simulink model "IEEE34_SPSload"  (R2021b)
settings: Solver=ode4  StartTime=0.0  StopTime=5  FixedStep=50e-6  RelTol=1e-3
PreLoadFcn:
  | pGain = 0.05; % Gain of random perturbation (pu)
  | pGainAP = 0.01; % Gain of sinusoidal active power variation (pu)
  | pGainRP = 0.01; % Gain of sinusoidal reactive power variation (pu)
  | pFreqAP = 0.03; % Frequency of sinusoidal active power variation (Hz)
  | pFreqRP = 0.03; % Frequency of sinusoidal reactive power variation (Hz)
  | 
  | init_IEEE34nodetestfeeder;
InitFcn:
  | pGain = 0.05; % Gain of random perturbation (pu)
  | pGainAP = 0.01; % Gain of sinusoidal active power variation (pu)
  | pGainRP = 0.01; % Gain of sinusoidal reactive power variation (pu)
  | pFreqAP = 0.03; % Frequency of sinusoidal active power variation (Hz)
  | pFreqRP = 0.03; % Frequency of sinusoidal reactive power variation (Hz)
  | 
  | init_IEEE34nodetestfeeder;
values from neighbouring files (symbols this model uses):
  fNom = f    (= 60)    [init_IEEE34nodetestfeeder.m]
  loadcoeff = 1.0    (= 1)    [init_IEEE34nodetestfeeder.m]
  Ts = 50e-6    (= 5e-05)    [init_IEEE34nodetestfeeder.m]
  vNomMV = VsubL    (= 24900)    [init_IEEE34nodetestfeeder.m]
  VsubL = 24.9e3    (= 24900)    [init_IEEE34nodetestfeeder.m]
  VxfmL = 4.16e3    (= 4160)    [init_IEEE34nodetestfeeder.m]
undefined symbols (not defined in the file or in its folder): Ac, Bc, Cc, Dc, find_system, j
libraries: spsSeriesRLCBranchLib x418, spsGroundLib x242, simulink_extras x176, spsVoltageMeasurementLib x106, spsRMSLib x96, spsControlledCurrentSourceLib x94, spsThreePhaseVIMeasurementLib x37, spsMutualInductanceLib x24, spsCurrentMeasurementLib x12, spsOnDelayLib x12, spsLinearTransformerLib x6, spsControlledVoltageSourceLib x6
(part 18 of 33)

== system IEEE34_SPSload/SM_IEEE34/DL_802-1/Load B1/model/PLL ==
  v (pu) : Inport
  freq (pu) : Inport  Port=2
  Gain : Gain  Gain=2*pi
  Gain1 : Gain  Gain=500
  Gain2 : Gain  Gain=freq
  IC : InitialCondition
  Integrator : Integrator
  Integrator1 : Integrator
  Product : Product  Inputs=**  RndMeth=Zero
  Sum1 : Sum  InputSameDT=on  SaturateOnIntegerOverflow=on  OutDataTypeStr=Inherit: Same as first input
  Trigonometric Function : Trigonometry  Operator=cos
  adaptive filter : Subsystem
  adaptive mean : Subsystem
  alpha (rad) : Outport  VectorParamsAs1DForOutWhenUnconnected=off
  wt : Outport  Port=2  VectorParamsAs1DForOutWhenUnconnected=off
  wires:
  freq (pu)/1 -> Gain2/1
  Gain2/1 -> adaptive filter/2(freq (Hz)), adaptive mean/2(freq (Hz)), Gain/1
  Trigonometric Function/1 -> Product/2
  adaptive mean/1(y) -> alpha (rad)/1
  Integrator1/1 -> Gain1/1
  Gain1/1 -> Sum1/1, adaptive mean/1(u)
  Sum1/1 -> Trigonometric Function/1
  Integrator/1 -> Sum1/2, wt/1
  Gain/1 -> Integrator/1
  adaptive filter/1(y) -> Integrator1/1
  Product/1 -> adaptive filter/1(u)
  v (pu)/1 -> IC/1
  IC/1 -> Product/1

== system IEEE34_SPSload/SM_IEEE34/DL_802-1/Load B1/model/Positive Sequence current ==
  note: kp=Vmin^(np-2)/Vo^np
      | kq=Vmin^(nq-2)/Vo^nq
  note: V<Vmin
      | Constant impedance load :
      |
      |  P=Po*kp*V^2
      | Q=Qo*kq*V^2
  note: V>Vmin :
      |
      |    P=Po*(V/Vo)^np
      |    Q=Qo*(V/Vo)^np
  note: I1= (S/V1)'
  V1(pu) : Inport
  S_ext : Inport  Port=2
  Complex to Magnitude-Angle : ComplexToMagnitudeAngle  Output=Magnitude
  Complex to Real-Imag1 : ComplexToRealImag
  Conj1 : Math  Operator=conj  SignedPower=on  SaturateOnIntegerOverflow=on
  Math Function : Math  Operator=square  SignedPower=on  SaturateOnIntegerOverflow=on
  Mux1 : Mux  Inputs=3
  Mux2 : Mux  Inputs=2
  Mux3 : Mux  Inputs=2
  P0/ (Vo^np) : Gain  Gain=P0/(Mag_V0^np)  SaturateOnIntegerOverflow=on  OutDataTypeStr=Inherit: Same as input  ParamDataTypeStr=Inherit: Same as input
  PQ_ext : Constant  Value=PQext
  Product : Product  Inputs=/*  InputSameDT=on  SaturateOnIntegerOverflow=on  OutDataTypeStr=Inherit: Same as first input
  Q0/(Vo^nq) : Gain  Gain=Q0/(Mag_V0^nq)  SaturateOnIntegerOverflow=on  OutDataTypeStr=Inherit: Same as input  ParamDataTypeStr=Inherit: Same as input
  Real-Imag to Complex : RealImagToComplex
  Switch1 : Switch  Threshold=0.5  InputSameDT=on
  Switch3 : Switch  Threshold=Vmin  InputSameDT=on
  Switch4 : Switch  Threshold=Vmin  InputSameDT=on
  TF_P : Subsystem  mask(Transfer function){T1=Tp1, T2=Tp2, V_Init=P0}
      mask prompts: T1 "Time constant T1 (s):"; T2 "Time constant T2 (s):"; V_Init "Initial input and output :"
      mask help:
      | This block implements a continuous transfer function:
      |
      |          1+T1s
      | H(s)= ------
      |          1+T2s
      |
      | States are initialized according to  initial input and output value so that simulation starts in steady state.
      mask init:
      | numc=[T1 1];
      | denc=[T2 1];
      | [Ac,Bc,Cc,Dc]=tf2ss(numc,denc);
      | 
      | % Compute Initial states
      | I=eye(size(Ac));
      | x0c=inv(-Ac)*Bc*V_Init;
      mask Display: disp('1+T1s\n---\n1+T2s')
  TF_Q : Subsystem  mask(Transfer function){T1=Tq1, T2=Tq2, V_Init=Q0}
      mask prompts: T1 "Time constant T1 (s):"; T2 "Time constant T2 (s):"; V_Init "Initial input and output :"
      mask help:
      | This block implements a continuous transfer function:
      |
      |          1+T1s
      | H(s)= ------
      |          1+T2s
      |
      | States are initialized according to  initial input and output value so that simulation starts in steady state.
      mask init:
      | numc=[T1 1];
      | denc=[T2 1];
      | [Ac,Bc,Cc,Dc]=tf2ss(numc,denc);
      | 
      | % Compute Initial states
      | I=eye(size(Ac));
      | x0c=inv(-Ac)*Bc*V_Init;
      mask Display: disp('1+T1s\n---\n1+T2s')
  V^nq : Fcn  Expr=u[1]^u[2]
  V^nq , : Fcn  Expr=u[1]^u[2]
  Vmin^(np-2) : Gain  Gain=Vmin^(np-2)  SaturateOnIntegerOverflow=on  OutDataTypeStr=Inherit: Same as input  ParamDataTypeStr=Inherit: Same as input
  Vmin^(nq-2) : Gain  Gain=Vmin^(nq-2)  SaturateOnIntegerOverflow=on  OutDataTypeStr=Inherit: Same as input  ParamDataTypeStr=Inherit: Same as input
  np : Constant  Value=np
  nq : Constant  Value=nq
  pu>V : Gain  Gain=Vnom/sqrt(2)  SaturateOnIntegerOverflow=on  OutDataTypeStr=Inherit: Same as input  ParamDataTypeStr=Inherit: Same as input
  I1(A) : Outport  VectorParamsAs1DForOutWhenUnconnected=off
  VPQ : Outport  Port=2  VectorParamsAs1DForOutWhenUnconnected=off
  wires:
  Vmin^(nq-2)/1 -> Switch4/3
  V^nq ,/1 -> Switch3/1
  Vmin^(np-2)/1 -> Switch3/3
  Math Function/1 -> Vmin^(nq-2)/1, Vmin^(np-2)/1
  V^nq/1 -> Switch4/1
  V1(pu)/1 -> Complex to Magnitude-Angle/1, pu>V/1
  Mux3/1 -> V^nq/1
  nq/1 -> Mux3/2
  Mux2/1 -> V^nq ,/1
  np/1 -> Mux2/2
  Switch3/1 -> P0/ (Vo^np)/1
  Q0/(Vo^nq)/1 -> TF_Q/1(In1)
  P0/ (Vo^np)/1 -> TF_P/1(In1)
  Switch4/1 -> Q0/(Vo^nq)/1
  Product/1 -> Conj1/1
  Conj1/1 -> I1(A)/1
  Switch1/1 -> Product/2, Complex to Real-Imag1/1  "S=P+jQ"
  Real-Imag to Complex/1 -> Switch1/3  "S_dyn"
  S_ext/1 -> Switch1/1
  PQ_ext/1 -> Switch1/2
  pu>V/1 -> Product/1
  Complex to Magnitude-Angle/1 -> Math Function/1, Mux3/1, Mux2/1, Switch3/2, Switch4/2, Mux1/1
  Mux1/1 -> VPQ/1
  Complex to Real-Imag1/1 -> Mux1/2
  Complex to Real-Imag1/2 -> Mux1/3
  TF_P/1(Out1) -> Real-Imag to Complex/1
  TF_Q/1(Out1) -> Real-Imag to Complex/2

== system IEEE34_SPSload/SM_IEEE34/DL_802-1/Load C/model/Break Alg. Loop ==
  In : Inport
  Complex to Real-Imag : ComplexToRealImag
  Real-Imag to Complex : RealImagToComplex
  imag : simulink_extras/Additional Linear/Transfer Fcn (with initial outputs)  N=[1]  D="[100e-6  1]"  Y0=imag(I1_init*exp(-j*Pha_V0*pi/180))  U0=imag(I1_init*exp(-j*Pha_V0*pi/180))
  real : simulink_extras/Additional Linear/Transfer Fcn (with initial outputs)  N=[1]  D="[100e-6  1]"  Y0=real(I1_init*exp(-j*Pha_V0*pi/180))  U0=real(I1_init*exp(-j*Pha_V0*pi/180))
  Out : Outport  VectorParamsAs1DForOutWhenUnconnected=off
  wires:
  imag/1 -> Real-Imag to Complex/2
  Complex to Real-Imag/2 -> imag/1
  real/1 -> Real-Imag to Complex/1
  Complex to Real-Imag/1 -> real/1
  Real-Imag to Complex/1 -> Out/1
  In/1 -> Complex to Real-Imag/1

== system IEEE34_SPSload/SM_IEEE34/DL_802-1/Load C/model/PLL ==
  v (pu) : Inport
  freq (pu) : Inport  Port=2
  Gain : Gain  Gain=2*pi
  Gain1 : Gain  Gain=500
  Gain2 : Gain  Gain=freq
  IC : InitialCondition
  Integrator : Integrator
  Integrator1 : Integrator
  Product : Product  Inputs=**  RndMeth=Zero
  Sum1 : Sum  InputSameDT=on  SaturateOnIntegerOverflow=on  OutDataTypeStr=Inherit: Same as first input
  Trigonometric Function : Trigonometry  Operator=cos
  adaptive filter : Subsystem
  adaptive mean : Subsystem
  alpha (rad) : Outport  VectorParamsAs1DForOutWhenUnconnected=off
  wt : Outport  Port=2  VectorParamsAs1DForOutWhenUnconnected=off
  wires:
  freq (pu)/1 -> Gain2/1
  Gain2/1 -> adaptive filter/2(freq (Hz)), adaptive mean/2(freq (Hz)), Gain/1
  Trigonometric Function/1 -> Product/2
  adaptive mean/1(y) -> alpha (rad)/1
  Integrator1/1 -> Gain1/1
  Gain1/1 -> Sum1/1, adaptive mean/1(u)
  Sum1/1 -> Trigonometric Function/1
  Integrator/1 -> Sum1/2, wt/1
  Gain/1 -> Integrator/1
  adaptive filter/1(y) -> Integrator1/1
  Product/1 -> adaptive filter/1(u)
  v (pu)/1 -> IC/1
  IC/1 -> Product/1

== system IEEE34_SPSload/SM_IEEE34/DL_802-1/Load C/model/Positive Sequence current ==
  note: kp=Vmin^(np-2)/Vo^np
      | kq=Vmin^(nq-2)/Vo^nq
  note: V<Vmin
      | Constant impedance load :
      |
      |  P=Po*kp*V^2
      | Q=Qo*kq*V^2
  note: V>Vmin :
      |
      |    P=Po*(V/Vo)^np
      |    Q=Qo*(V/Vo)^np
  note: I1= (S/V1)'
  V1(pu) : Inport
  S_ext : Inport  Port=2
  Complex to Magnitude-Angle : ComplexToMagnitudeAngle  Output=Magnitude
  Complex to Real-Imag1 : ComplexToRealImag
  Conj1 : Math  Operator=conj  SignedPower=on  SaturateOnIntegerOverflow=on
  Math Function : Math  Operator=square  SignedPower=on  SaturateOnIntegerOverflow=on
  Mux1 : Mux  Inputs=3
  Mux2 : Mux  Inputs=2
  Mux3 : Mux  Inputs=2
  P0/ (Vo^np) : Gain  Gain=P0/(Mag_V0^np)  SaturateOnIntegerOverflow=on  OutDataTypeStr=Inherit: Same as input  ParamDataTypeStr=Inherit: Same as input
  PQ_ext : Constant  Value=PQext
  Product : Product  Inputs=/*  InputSameDT=on  SaturateOnIntegerOverflow=on  OutDataTypeStr=Inherit: Same as first input
  Q0/(Vo^nq) : Gain  Gain=Q0/(Mag_V0^nq)  SaturateOnIntegerOverflow=on  OutDataTypeStr=Inherit: Same as input  ParamDataTypeStr=Inherit: Same as input
  Real-Imag to Complex : RealImagToComplex
  Switch1 : Switch  Threshold=0.5  InputSameDT=on
  Switch3 : Switch  Threshold=Vmin  InputSameDT=on
  Switch4 : Switch  Threshold=Vmin  InputSameDT=on
  TF_P : Subsystem  mask(Transfer function){T1=Tp1, T2=Tp2, V_Init=P0}
      mask prompts: T1 "Time constant T1 (s):"; T2 "Time constant T2 (s):"; V_Init "Initial input and output :"
      mask help:
      | This block implements a continuous transfer function:
      |
      |          1+T1s
      | H(s)= ------
      |          1+T2s
      |
      | States are initialized according to  initial input and output value so that simulation starts in steady state.
      mask init:
      | numc=[T1 1];
      | denc=[T2 1];
      | [Ac,Bc,Cc,Dc]=tf2ss(numc,denc);
      | 
      | % Compute Initial states
      | I=eye(size(Ac));
      | x0c=inv(-Ac)*Bc*V_Init;
      mask Display: disp('1+T1s\n---\n1+T2s')
  TF_Q : Subsystem  mask(Transfer function){T1=Tq1, T2=Tq2, V_Init=Q0}
      mask prompts: T1 "Time constant T1 (s):"; T2 "Time constant T2 (s):"; V_Init "Initial input and output :"
      mask help:
      | This block implements a continuous transfer function:
      |
      |          1+T1s
      | H(s)= ------
      |          1+T2s
      |
      | States are initialized according to  initial input and output value so that simulation starts in steady state.
      mask init:
      | numc=[T1 1];
      | denc=[T2 1];
      | [Ac,Bc,Cc,Dc]=tf2ss(numc,denc);
      | 
      | % Compute Initial states
      | I=eye(size(Ac));
      | x0c=inv(-Ac)*Bc*V_Init;
      mask Display: disp('1+T1s\n---\n1+T2s')
  V^nq : Fcn  Expr=u[1]^u[2]
  V^nq , : Fcn  Expr=u[1]^u[2]
  Vmin^(np-2) : Gain  Gain=Vmin^(np-2)  SaturateOnIntegerOverflow=on  OutDataTypeStr=Inherit: Same as input  ParamDataTypeStr=Inherit: Same as input
  Vmin^(nq-2) : Gain  Gain=Vmin^(nq-2)  SaturateOnIntegerOverflow=on  OutDataTypeStr=Inherit: Same as input  ParamDataTypeStr=Inherit: Same as input
  np : Constant  Value=np
  nq : Constant  Value=nq
  pu>V : Gain  Gain=Vnom/sqrt(2)  SaturateOnIntegerOverflow=on  OutDataTypeStr=Inherit: Same as input  ParamDataTypeStr=Inherit: Same as input
  I1(A) : Outport  VectorParamsAs1DForOutWhenUnconnected=off
  VPQ : Outport  Port=2  VectorParamsAs1DForOutWhenUnconnected=off
  wires:
  Vmin^(nq-2)/1 -> Switch4/3
  V^nq ,/1 -> Switch3/1
  Vmin^(np-2)/1 -> Switch3/3
  Math Function/1 -> Vmin^(nq-2)/1, Vmin^(np-2)/1
  V^nq/1 -> Switch4/1
  V1(pu)/1 -> Complex to Magnitude-Angle/1, pu>V/1
  Mux3/1 -> V^nq/1
  nq/1 -> Mux3/2
  Mux2/1 -> V^nq ,/1
  np/1 -> Mux2/2
  Switch3/1 -> P0/ (Vo^np)/1
  Q0/(Vo^nq)/1 -> TF_Q/1(In1)
  P0/ (Vo^np)/1 -> TF_P/1(In1)
  Switch4/1 -> Q0/(Vo^nq)/1
  Product/1 -> Conj1/1
  Conj1/1 -> I1(A)/1
  Switch1/1 -> Product/2, Complex to Real-Imag1/1  "S=P+jQ"
  Real-Imag to Complex/1 -> Switch1/3  "S_dyn"
  S_ext/1 -> Switch1/1
  PQ_ext/1 -> Switch1/2
  pu>V/1 -> Product/1
  Complex to Magnitude-Angle/1 -> Math Function/1, Mux3/1, Mux2/1, Switch3/2, Switch4/2, Mux1/1
  Mux1/1 -> VPQ/1
  Complex to Real-Imag1/1 -> Mux1/2
  Complex to Real-Imag1/2 -> Mux1/3
  TF_P/1(Out1) -> Real-Imag to Complex/1
  TF_Q/1(Out1) -> Real-Imag to Complex/2

== system IEEE34_SPSload/SM_IEEE34/DL_802-2/Load B/model/Break Alg. Loop ==
  In : Inport
  Complex to Real-Imag : ComplexToRealImag
  Real-Imag to Complex : RealImagToComplex
  imag : simulink_extras/Additional Linear/Transfer Fcn (with initial outputs)  N=[1]  D="[100e-6  1]"  Y0=imag(I1_init*exp(-j*Pha_V0*pi/180))  U0=imag(I1_init*exp(-j*Pha_V0*pi/180))
  real : simulink_extras/Additional Linear/Transfer Fcn (with initial outputs)  N=[1]  D="[100e-6  1]"  Y0=real(I1_init*exp(-j*Pha_V0*pi/180))  U0=real(I1_init*exp(-j*Pha_V0*pi/180))
  Out : Outport  VectorParamsAs1DForOutWhenUnconnected=off
  wires:
  imag/1 -> Real-Imag to Complex/2
  Complex to Real-Imag/2 -> imag/1
  real/1 -> Real-Imag to Complex/1
  Complex to Real-Imag/1 -> real/1
  Real-Imag to Complex/1 -> Out/1
  In/1 -> Complex to Real-Imag/1

== system IEEE34_SPSload/SM_IEEE34/DL_802-2/Load B/model/PLL ==
  v (pu) : Inport
  freq (pu) : Inport  Port=2
  Gain : Gain  Gain=2*pi
  Gain1 : Gain  Gain=500
  Gain2 : Gain  Gain=freq
  IC : InitialCondition
  Integrator : Integrator
  Integrator1 : Integrator
  Product : Product  Inputs=**  RndMeth=Zero
  Sum1 : Sum  InputSameDT=on  SaturateOnIntegerOverflow=on  OutDataTypeStr=Inherit: Same as first input
  Trigonometric Function : Trigonometry  Operator=cos
  adaptive filter : Subsystem
  adaptive mean : Subsystem
  alpha (rad) : Outport  VectorParamsAs1DForOutWhenUnconnected=off
  wt : Outport  Port=2  VectorParamsAs1DForOutWhenUnconnected=off
  wires:
  freq (pu)/1 -> Gain2/1
  Gain2/1 -> adaptive filter/2(freq (Hz)), adaptive mean/2(freq (Hz)), Gain/1
  Trigonometric Function/1 -> Product/2
  adaptive mean/1(y) -> alpha (rad)/1
  Integrator1/1 -> Gain1/1
  Gain1/1 -> Sum1/1, adaptive mean/1(u)
  Sum1/1 -> Trigonometric Function/1
  Integrator/1 -> Sum1/2, wt/1
  Gain/1 -> Integrator/1
  adaptive filter/1(y) -> Integrator1/1
  Product/1 -> adaptive filter/1(u)
  v (pu)/1 -> IC/1
  IC/1 -> Product/1

== system IEEE34_SPSload/SM_IEEE34/DL_802-2/Load B/model/Positive Sequence current ==
  note: kp=Vmin^(np-2)/Vo^np
      | kq=Vmin^(nq-2)/Vo^nq
  note: V<Vmin
      | Constant impedance load :
      |
      |  P=Po*kp*V^2
      | Q=Qo*kq*V^2
  note: V>Vmin :
      |
      |    P=Po*(V/Vo)^np
      |    Q=Qo*(V/Vo)^np
  note: I1= (S/V1)'
  V1(pu) : Inport
  S_ext : Inport  Port=2
  Complex to Magnitude-Angle : ComplexToMagnitudeAngle  Output=Magnitude
  Complex to Real-Imag1 : ComplexToRealImag
  Conj1 : Math  Operator=conj  SignedPower=on  SaturateOnIntegerOverflow=on
  Math Function : Math  Operator=square  SignedPower=on  SaturateOnIntegerOverflow=on
  Mux1 : Mux  Inputs=3
  Mux2 : Mux  Inputs=2
  Mux3 : Mux  Inputs=2
  P0/ (Vo^np) : Gain  Gain=P0/(Mag_V0^np)  SaturateOnIntegerOverflow=on  OutDataTypeStr=Inherit: Same as input  ParamDataTypeStr=Inherit: Same as input
  PQ_ext : Constant  Value=PQext
  Product : Product  Inputs=/*  InputSameDT=on  SaturateOnIntegerOverflow=on  OutDataTypeStr=Inherit: Same as first input
  Q0/(Vo^nq) : Gain  Gain=Q0/(Mag_V0^nq)  SaturateOnIntegerOverflow=on  OutDataTypeStr=Inherit: Same as input  ParamDataTypeStr=Inherit: Same as input
  Real-Imag to Complex : RealImagToComplex
  Switch1 : Switch  Threshold=0.5  InputSameDT=on
  Switch3 : Switch  Threshold=Vmin  InputSameDT=on
  Switch4 : Switch  Threshold=Vmin  InputSameDT=on
  TF_P : Subsystem  mask(Transfer function){T1=Tp1, T2=Tp2, V_Init=P0}
      mask prompts: T1 "Time constant T1 (s):"; T2 "Time constant T2 (s):"; V_Init "Initial input and output :"
      mask help:
      | This block implements a continuous transfer function:
      |
      |          1+T1s
      | H(s)= ------
      |          1+T2s
      |
      | States are initialized according to  initial input and output value so that simulation starts in steady state.
      mask init:
      | numc=[T1 1];
      | denc=[T2 1];
      | [Ac,Bc,Cc,Dc]=tf2ss(numc,denc);
      | 
      | % Compute Initial states
      | I=eye(size(Ac));
      | x0c=inv(-Ac)*Bc*V_Init;
      mask Display: disp('1+T1s\n---\n1+T2s')
  TF_Q : Subsystem  mask(Transfer function){T1=Tq1, T2=Tq2, V_Init=Q0}
      mask prompts: T1 "Time constant T1 (s):"; T2 "Time constant T2 (s):"; V_Init "Initial input and output :"
      mask help:
      | This block implements a continuous transfer function:
      |
      |          1+T1s
      | H(s)= ------
      |          1+T2s
      |
      | States are initialized according to  initial input and output value so that simulation starts in steady state.
      mask init:
      | numc=[T1 1];
      | denc=[T2 1];
      | [Ac,Bc,Cc,Dc]=tf2ss(numc,denc);
      | 
      | % Compute Initial states
      | I=eye(size(Ac));
      | x0c=inv(-Ac)*Bc*V_Init;
      mask Display: disp('1+T1s\n---\n1+T2s')
  V^nq : Fcn  Expr=u[1]^u[2]
  V^nq , : Fcn  Expr=u[1]^u[2]
  Vmin^(np-2) : Gain  Gain=Vmin^(np-2)  SaturateOnIntegerOverflow=on  OutDataTypeStr=Inherit: Same as input  ParamDataTypeStr=Inherit: Same as input
  Vmin^(nq-2) : Gain  Gain=Vmin^(nq-2)  SaturateOnIntegerOverflow=on  OutDataTypeStr=Inherit: Same as input  ParamDataTypeStr=Inherit: Same as input
  np : Constant  Value=np
  nq : Constant  Value=nq
  pu>V : Gain  Gain=Vnom/sqrt(2)  SaturateOnIntegerOverflow=on  OutDataTypeStr=Inherit: Same as input  ParamDataTypeStr=Inherit: Same as input
  I1(A) : Outport  VectorParamsAs1DForOutWhenUnconnected=off
  VPQ : Outport  Port=2  VectorParamsAs1DForOutWhenUnconnected=off
  wires:
  Vmin^(nq-2)/1 -> Switch4/3
  V^nq ,/1 -> Switch3/1
  Vmin^(np-2)/1 -> Switch3/3
  Math Function/1 -> Vmin^(nq-2)/1, Vmin^(np-2)/1
  V^nq/1 -> Switch4/1
  V1(pu)/1 -> Complex to Magnitude-Angle/1, pu>V/1
  Mux3/1 -> V^nq/1
  nq/1 -> Mux3/2
  Mux2/1 -> V^nq ,/1
  np/1 -> Mux2/2
  Switch3/1 -> P0/ (Vo^np)/1
  Q0/(Vo^nq)/1 -> TF_Q/1(In1)
  P0/ (Vo^np)/1 -> TF_P/1(In1)
  Switch4/1 -> Q0/(Vo^nq)/1
  Product/1 -> Conj1/1
  Conj1/1 -> I1(A)/1
  Switch1/1 -> Product/2, Complex to Real-Imag1/1  "S=P+jQ"
  Real-Imag to Complex/1 -> Switch1/3  "S_dyn"
  S_ext/1 -> Switch1/1
  PQ_ext/1 -> Switch1/2
  pu>V/1 -> Product/1
  Complex to Magnitude-Angle/1 -> Math Function/1, Mux3/1, Mux2/1, Switch3/2, Switch4/2, Mux1/1
  Mux1/1 -> VPQ/1
  Complex to Real-Imag1/1 -> Mux1/2
  Complex to Real-Imag1/2 -> Mux1/3
  TF_P/1(Out1) -> Real-Imag to Complex/1
  TF_Q/1(Out1) -> Real-Imag to Complex/2

== system IEEE34_SPSload/SM_IEEE34/DL_802-2/Load B1/model/Break Alg. Loop ==
  In : Inport
  Complex to Real-Imag : ComplexToRealImag
  Real-Imag to Complex : RealImagToComplex
  imag : simulink_extras/Additional Linear/Transfer Fcn (with initial outputs)  N=[1]  D="[100e-6  1]"  Y0=imag(I1_init*exp(-j*Pha_V0*pi/180))  U0=imag(I1_init*exp(-j*Pha_V0*pi/180))
  real : simulink_extras/Additional Linear/Transfer Fcn (with initial outputs)  N=[1]  D="[100e-6  1]"  Y0=real(I1_init*exp(-j*Pha_V0*pi/180))  U0=real(I1_init*exp(-j*Pha_V0*pi/180))
  Out : Outport  VectorParamsAs1DForOutWhenUnconnected=off
  wires:
  In/1 -> Complex to Real-Imag/1
  Real-Imag to Complex/1 -> Out/1
  Complex to Real-Imag/1 -> real/1
  real/1 -> Real-Imag to Complex/1
  Complex to Real-Imag/2 -> imag/1
  imag/1 -> Real-Imag to Complex/2

== system IEEE34_SPSload/SM_IEEE34/DL_802-2/Load B1/model/PLL ==
  v (pu) : Inport
  freq (pu) : Inport  Port=2
  Gain : Gain  Gain=2*pi
  Gain1 : Gain  Gain=500
  Gain2 : Gain  Gain=freq
  IC : InitialCondition
  Integrator : Integrator
  Integrator1 : Integrator
  Product : Product  Inputs=**  RndMeth=Zero
  Sum1 : Sum  InputSameDT=on  SaturateOnIntegerOverflow=on  OutDataTypeStr=Inherit: Same as first input
  Trigonometric Function : Trigonometry  Operator=cos
  adaptive filter : Subsystem
  adaptive mean : Subsystem
  alpha (rad) : Outport  VectorParamsAs1DForOutWhenUnconnected=off
  wt : Outport  Port=2  VectorParamsAs1DForOutWhenUnconnected=off
  wires:
  IC/1 -> Product/1
  v (pu)/1 -> IC/1
  Product/1 -> adaptive filter/1(u)
  adaptive filter/1(y) -> Integrator1/1
  Gain/1 -> Integrator/1
  Integrator/1 -> wt/1, Sum1/2
  Sum1/1 -> Trigonometric Function/1
  Gain1/1 -> adaptive mean/1(u), Sum1/1
  Integrator1/1 -> Gain1/1
  adaptive mean/1(y) -> alpha (rad)/1
  Trigonometric Function/1 -> Product/2
  Gain2/1 -> Gain/1, adaptive mean/2(freq (Hz)), adaptive filter/2(freq (Hz))
  freq (pu)/1 -> Gain2/1

== system IEEE34_SPSload/SM_IEEE34/DL_802-2/Load B1/model/Positive Sequence current ==
  note: I1= (S/V1)'
  note: V>Vmin :
      |
      |    P=Po*(V/Vo)^np
      |    Q=Qo*(V/Vo)^np
  note: V<Vmin
      | Constant impedance load :
      |
      |  P=Po*kp*V^2
      | Q=Qo*kq*V^2
  note: kp=Vmin^(np-2)/Vo^np
      | kq=Vmin^(nq-2)/Vo^nq
  V1(pu) : Inport
  S_ext : Inport  Port=2
  Complex to Magnitude-Angle : ComplexToMagnitudeAngle  Output=Magnitude
  Complex to Real-Imag1 : ComplexToRealImag
  Conj1 : Math  Operator=conj  SignedPower=on  SaturateOnIntegerOverflow=on
  Math Function : Math  Operator=square  SignedPower=on  SaturateOnIntegerOverflow=on
  Mux1 : Mux  Inputs=3
  Mux2 : Mux  Inputs=2
  Mux3 : Mux  Inputs=2
  P0/ (Vo^np) : Gain  Gain=P0/(Mag_V0^np)  SaturateOnIntegerOverflow=on  OutDataTypeStr=Inherit: Same as input  ParamDataTypeStr=Inherit: Same as input
  PQ_ext : Constant  Value=PQext
  Product : Product  Inputs=/*  InputSameDT=on  SaturateOnIntegerOverflow=on  OutDataTypeStr=Inherit: Same as first input
  Q0/(Vo^nq) : Gain  Gain=Q0/(Mag_V0^nq)  SaturateOnIntegerOverflow=on  OutDataTypeStr=Inherit: Same as input  ParamDataTypeStr=Inherit: Same as input
  Real-Imag to Complex : RealImagToComplex
  Switch1 : Switch  Threshold=0.5  InputSameDT=on
  Switch3 : Switch  Threshold=Vmin  InputSameDT=on
  Switch4 : Switch  Threshold=Vmin  InputSameDT=on
  TF_P : Subsystem  mask(Transfer function){T1=Tp1, T2=Tp2, V_Init=P0}
      mask prompts: T1 "Time constant T1 (s):"; T2 "Time constant T2 (s):"; V_Init "Initial input and output :"
      mask help:
      | This block implements a continuous transfer function:
      |
      |          1+T1s
      | H(s)= ------
      |          1+T2s
      |
      | States are initialized according to  initial input and output value so that simulation starts in steady state.
      mask init:
      | numc=[T1 1];
      | denc=[T2 1];
      | [Ac,Bc,Cc,Dc]=tf2ss(numc,denc);
      | 
      | % Compute Initial states
      | I=eye(size(Ac));
      | x0c=inv(-Ac)*Bc*V_Init;
      mask Display: disp('1+T1s\n---\n1+T2s')
  TF_Q : Subsystem  mask(Transfer function){T1=Tq1, T2=Tq2, V_Init=Q0}
      mask prompts: T1 "Time constant T1 (s):"; T2 "Time constant T2 (s):"; V_Init "Initial input and output :"
      mask help:
      | This block implements a continuous transfer function:
      |
      |          1+T1s
      | H(s)= ------
      |          1+T2s
      |
      | States are initialized according to  initial input and output value so that simulation starts in steady state.
      mask init:
      | numc=[T1 1];
      | denc=[T2 1];
      | [Ac,Bc,Cc,Dc]=tf2ss(numc,denc);
      | 
      | % Compute Initial states
      | I=eye(size(Ac));
      | x0c=inv(-Ac)*Bc*V_Init;
      mask Display: disp('1+T1s\n---\n1+T2s')
  V^nq : Fcn  Expr=u[1]^u[2]
  V^nq , : Fcn  Expr=u[1]^u[2]
  Vmin^(np-2) : Gain  Gain=Vmin^(np-2)  SaturateOnIntegerOverflow=on  OutDataTypeStr=Inherit: Same as input  ParamDataTypeStr=Inherit: Same as input
  Vmin^(nq-2) : Gain  Gain=Vmin^(nq-2)  SaturateOnIntegerOverflow=on  OutDataTypeStr=Inherit: Same as input  ParamDataTypeStr=Inherit: Same as input
  np : Constant  Value=np
  nq : Constant  Value=nq
  pu>V : Gain  Gain=Vnom/sqrt(2)  SaturateOnIntegerOverflow=on  OutDataTypeStr=Inherit: Same as input  ParamDataTypeStr=Inherit: Same as input
  I1(A) : Outport  VectorParamsAs1DForOutWhenUnconnected=off
  VPQ : Outport  Port=2  VectorParamsAs1DForOutWhenUnconnected=off
  wires:
  TF_Q/1(Out1) -> Real-Imag to Complex/2
  TF_P/1(Out1) -> Real-Imag to Complex/1
  Complex to Real-Imag1/2 -> Mux1/3
  Complex to Real-Imag1/1 -> Mux1/2
  Mux1/1 -> VPQ/1
  Complex to Magnitude-Angle/1 -> Mux1/1, Switch4/2, Switch3/2, Mux2/1, Mux3/1, Math Function/1
  pu>V/1 -> Product/1
  PQ_ext/1 -> Switch1/2
  S_ext/1 -> Switch1/1
  Real-Imag to Complex/1 -> Switch1/3  "S_dyn"
  Switch1/1 -> Complex to Real-Imag1/1, Product/2  "S=P+jQ"
  Conj1/1 -> I1(A)/1
  Product/1 -> Conj1/1
  Switch4/1 -> Q0/(Vo^nq)/1
  P0/ (Vo^np)/1 -> TF_P/1(In1)
  Q0/(Vo^nq)/1 -> TF_Q/1(In1)
  Switch3/1 -> P0/ (Vo^np)/1
  np/1 -> Mux2/2
  Mux2/1 -> V^nq ,/1
  nq/1 -> Mux3/2
  Mux3/1 -> V^nq/1
  V1(pu)/1 -> pu>V/1, Complex to Magnitude-Angle/1
  V^nq/1 -> Switch4/1
  Math Function/1 -> Vmin^(np-2)/1, Vmin^(nq-2)/1
  Vmin^(np-2)/1 -> Switch3/3
  V^nq ,/1 -> Switch3/1
  Vmin^(nq-2)/1 -> Switch4/3

== system IEEE34_SPSload/SM_IEEE34/DL_802-2/Load C/model/Break Alg. Loop ==
  In : Inport
  Complex to Real-Imag : ComplexToRealImag
  Real-Imag to Complex : RealImagToComplex
  imag : simulink_extras/Additional Linear/Transfer Fcn (with initial outputs)  N=[1]  D="[100e-6  1]"  Y0=imag(I1_init*exp(-j*Pha_V0*pi/180))  U0=imag(I1_init*exp(-j*Pha_V0*pi/180))
  real : simulink_extras/Additional Linear/Transfer Fcn (with initial outputs)  N=[1]  D="[100e-6  1]"  Y0=real(I1_init*exp(-j*Pha_V0*pi/180))  U0=real(I1_init*exp(-j*Pha_V0*pi/180))
  Out : Outport  VectorParamsAs1DForOutWhenUnconnected=off
  wires:
  In/1 -> Complex to Real-Imag/1
  Real-Imag to Complex/1 -> Out/1
  Complex to Real-Imag/1 -> real/1
  real/1 -> Real-Imag to Complex/1
  Complex to Real-Imag/2 -> imag/1
  imag/1 -> Real-Imag to Complex/2

== system IEEE34_SPSload/SM_IEEE34/DL_802-2/Load C/model/PLL ==
  v (pu) : Inport
  freq (pu) : Inport  Port=2
  Gain : Gain  Gain=2*pi
  Gain1 : Gain  Gain=500
  Gain2 : Gain  Gain=freq
  IC : InitialCondition
  Integrator : Integrator
  Integrator1 : Integrator
  Product : Product  Inputs=**  RndMeth=Zero
  Sum1 : Sum  InputSameDT=on  SaturateOnIntegerOverflow=on  OutDataTypeStr=Inherit: Same as first input
  Trigonometric Function : Trigonometry  Operator=cos
  adaptive filter : Subsystem
  adaptive mean : Subsystem
  alpha (rad) : Outport  VectorParamsAs1DForOutWhenUnconnected=off
  wt : Outport  Port=2  VectorParamsAs1DForOutWhenUnconnected=off
  wires:
  IC/1 -> Product/1
  v (pu)/1 -> IC/1
  Product/1 -> adaptive filter/1(u)
  adaptive filter/1(y) -> Integrator1/1
  Gain/1 -> Integrator/1
  Integrator/1 -> wt/1, Sum1/2
  Sum1/1 -> Trigonometric Function/1
  Gain1/1 -> adaptive mean/1(u), Sum1/1
  Integrator1/1 -> Gain1/1
  adaptive mean/1(y) -> alpha (rad)/1
  Trigonometric Function/1 -> Product/2
  Gain2/1 -> Gain/1, adaptive mean/2(freq (Hz)), adaptive filter/2(freq (Hz))
  freq (pu)/1 -> Gain2/1

== system IEEE34_SPSload/SM_IEEE34/DL_802-2/Load C/model/Positive Sequence current ==
  note: I1= (S/V1)'
  note: V>Vmin :
      |
      |    P=Po*(V/Vo)^np
      |    Q=Qo*(V/Vo)^np
  note: V<Vmin
      | Constant impedance load :
      |
      |  P=Po*kp*V^2
      | Q=Qo*kq*V^2
  note: kp=Vmin^(np-2)/Vo^np
      | kq=Vmin^(nq-2)/Vo^nq
  V1(pu) : Inport
  S_ext : Inport  Port=2
  Complex to Magnitude-Angle : ComplexToMagnitudeAngle  Output=Magnitude
  Complex to Real-Imag1 : ComplexToRealImag
  Conj1 : Math  Operator=conj  SignedPower=on  SaturateOnIntegerOverflow=on
  Math Function : Math  Operator=square  SignedPower=on  SaturateOnIntegerOverflow=on
  Mux1 : Mux  Inputs=3
  Mux2 : Mux  Inputs=2
  Mux3 : Mux  Inputs=2
  P0/ (Vo^np) : Gain  Gain=P0/(Mag_V0^np)  SaturateOnIntegerOverflow=on  OutDataTypeStr=Inherit: Same as input  ParamDataTypeStr=Inherit: Same as input
  PQ_ext : Constant  Value=PQext
  Product : Product  Inputs=/*  InputSameDT=on  SaturateOnIntegerOverflow=on  OutDataTypeStr=Inherit: Same as first input
  Q0/(Vo^nq) : Gain  Gain=Q0/(Mag_V0^nq)  SaturateOnIntegerOverflow=on  OutDataTypeStr=Inherit: Same as input  ParamDataTypeStr=Inherit: Same as input
  Real-Imag to Complex : RealImagToComplex
  Switch1 : Switch  Threshold=0.5  InputSameDT=on
  Switch3 : Switch  Threshold=Vmin  InputSameDT=on
  Switch4 : Switch  Threshold=Vmin  InputSameDT=on
  TF_P : Subsystem  mask(Transfer function){T1=Tp1, T2=Tp2, V_Init=P0}
      mask prompts: T1 "Time constant T1 (s):"; T2 "Time constant T2 (s):"; V_Init "Initial input and output :"
      mask help:
      | This block implements a continuous transfer function:
      |
      |          1+T1s
      | H(s)= ------
      |          1+T2s
      |
      | States are initialized according to  initial input and output value so that simulation starts in steady state.
      mask init:
      | numc=[T1 1];
      | denc=[T2 1];
      | [Ac,Bc,Cc,Dc]=tf2ss(numc,denc);
      | 
      | % Compute Initial states
      | I=eye(size(Ac));
      | x0c=inv(-Ac)*Bc*V_Init;
      mask Display: disp('1+T1s\n---\n1+T2s')
  TF_Q : Subsystem  mask(Transfer function){T1=Tq1, T2=Tq2, V_Init=Q0}
      mask prompts: T1 "Time constant T1 (s):"; T2 "Time constant T2 (s):"; V_Init "Initial input and output :"
      mask help:
      | This block implements a continuous transfer function:
      |
      |          1+T1s
      | H(s)= ------
      |          1+T2s
      |
      | States are initialized according to  initial input and output value so that simulation starts in steady state.
      mask init:
      | numc=[T1 1];
      | denc=[T2 1];
      | [Ac,Bc,Cc,Dc]=tf2ss(numc,denc);
      | 
      | % Compute Initial states
      | I=eye(size(Ac));
      | x0c=inv(-Ac)*Bc*V_Init;
      mask Display: disp('1+T1s\n---\n1+T2s')
  V^nq : Fcn  Expr=u[1]^u[2]
  V^nq , : Fcn  Expr=u[1]^u[2]
  Vmin^(np-2) : Gain  Gain=Vmin^(np-2)  SaturateOnIntegerOverflow=on  OutDataTypeStr=Inherit: Same as input  ParamDataTypeStr=Inherit: Same as input
  Vmin^(nq-2) : Gain  Gain=Vmin^(nq-2)  SaturateOnIntegerOverflow=on  OutDataTypeStr=Inherit: Same as input  ParamDataTypeStr=Inherit: Same as input
  np : Constant  Value=np
  nq : Constant  Value=nq
  pu>V : Gain  Gain=Vnom/sqrt(2)  SaturateOnIntegerOverflow=on  OutDataTypeStr=Inherit: Same as input  ParamDataTypeStr=Inherit: Same as input
  I1(A) : Outport  VectorParamsAs1DForOutWhenUnconnected=off
  VPQ : Outport  Port=2  VectorParamsAs1DForOutWhenUnconnected=off
  wires:
  TF_Q/1(Out1) -> Real-Imag to Complex/2
  TF_P/1(Out1) -> Real-Imag to Complex/1
  Complex to Real-Imag1/2 -> Mux1/3
  Complex to Real-Imag1/1 -> Mux1/2
  Mux1/1 -> VPQ/1
  Complex to Magnitude-Angle/1 -> Mux1/1, Switch4/2, Switch3/2, Mux2/1, Mux3/1, Math Function/1
  pu>V/1 -> Product/1
  PQ_ext/1 -> Switch1/2
  S_ext/1 -> Switch1/1
  Real-Imag to Complex/1 -> Switch1/3  "S_dyn"
  Switch1/1 -> Complex to Real-Imag1/1, Product/2  "S=P+jQ"
  Conj1/1 -> I1(A)/1
  Product/1 -> Conj1/1
  Switch4/1 -> Q0/(Vo^nq)/1
  P0/ (Vo^np)/1 -> TF_P/1(In1)
  Q0/(Vo^nq)/1 -> TF_Q/1(In1)
  Switch3/1 -> P0/ (Vo^np)/1
  np/1 -> Mux2/2
  Mux2/1 -> V^nq ,/1
  nq/1 -> Mux3/2
  Mux3/1 -> V^nq/1
  V1(pu)/1 -> pu>V/1, Complex to Magnitude-Angle/1
  V^nq/1 -> Switch4/1
  Math Function/1 -> Vmin^(np-2)/1, Vmin^(nq-2)/1
  Vmin^(np-2)/1 -> Switch3/3
  V^nq ,/1 -> Switch3/1
  Vmin^(nq-2)/1 -> Switch4/3

== system IEEE34_SPSload/SM_IEEE34/DL_808-1/Load B/model/Break Alg. Loop ==
  In : Inport
  Complex to Real-Imag : ComplexToRealImag
  Real-Imag to Complex : RealImagToComplex
  imag : simulink_extras/Additional Linear/Transfer Fcn (with initial outputs)  N=[1]  D="[100e-6  1]"  Y0=imag(I1_init*exp(-j*Pha_V0*pi/180))  U0=imag(I1_init*exp(-j*Pha_V0*pi/180))
  real : simulink_extras/Additional Linear/Transfer Fcn (with initial outputs)  N=[1]  D="[100e-6  1]"  Y0=real(I1_init*exp(-j*Pha_V0*pi/180))  U0=real(I1_init*exp(-j*Pha_V0*pi/180))
  Out : Outport  VectorParamsAs1DForOutWhenUnconnected=off
  wires:
  In/1 -> Complex to Real-Imag/1
  Real-Imag to Complex/1 -> Out/1
  Complex to Real-Imag/1 -> real/1
  real/1 -> Real-Imag to Complex/1
  Complex to Real-Imag/2 -> imag/1
  imag/1 -> Real-Imag to Complex/2

== system IEEE34_SPSload/SM_IEEE34/DL_808-1/Load B/model/PLL ==
  v (pu) : Inport
  freq (pu) : Inport  Port=2
  Gain : Gain  Gain=2*pi
  Gain1 : Gain  Gain=500
  Gain2 : Gain  Gain=freq
  IC : InitialCondition
  Integrator : Integrator
  Integrator1 : Integrator
  Product : Product  Inputs=**  RndMeth=Zero
  Sum1 : Sum  InputSameDT=on  SaturateOnIntegerOverflow=on  OutDataTypeStr=Inherit: Same as first input
  Trigonometric Function : Trigonometry  Operator=cos
  adaptive filter : Subsystem
  adaptive mean : Subsystem
  alpha (rad) : Outport  VectorParamsAs1DForOutWhenUnconnected=off
  wt : Outport  Port=2  VectorParamsAs1DForOutWhenUnconnected=off
  wires:
  IC/1 -> Product/1
  v (pu)/1 -> IC/1
  Product/1 -> adaptive filter/1(u)
  adaptive filter/1(y) -> Integrator1/1
  Gain/1 -> Integrator/1
  Integrator/1 -> wt/1, Sum1/2
  Sum1/1 -> Trigonometric Function/1
  Gain1/1 -> adaptive mean/1(u), Sum1/1
  Integrator1/1 -> Gain1/1
  adaptive mean/1(y) -> alpha (rad)/1
  Trigonometric Function/1 -> Product/2
  Gain2/1 -> Gain/1, adaptive mean/2(freq (Hz)), adaptive filter/2(freq (Hz))
  freq (pu)/1 -> Gain2/1

== system IEEE34_SPSload/SM_IEEE34/DL_808-1/Load B/model/Positive Sequence current ==
  note: I1= (S/V1)'
  note: V>Vmin :
      |
      |    P=Po*(V/Vo)^np
      |    Q=Qo*(V/Vo)^np
  note: V<Vmin
      | Constant impedance load :
      |
      |  P=Po*kp*V^2
      | Q=Qo*kq*V^2
  note: kp=Vmin^(np-2)/Vo^np
      | kq=Vmin^(nq-2)/Vo^nq
  V1(pu) : Inport
  S_ext : Inport  Port=2
  Complex to Magnitude-Angle : ComplexToMagnitudeAngle  Output=Magnitude
  Complex to Real-Imag1 : ComplexToRealImag
  Conj1 : Math  Operator=conj  SignedPower=on  SaturateOnIntegerOverflow=on
  Math Function : Math  Operator=square  SignedPower=on  SaturateOnIntegerOverflow=on
  Mux1 : Mux  Inputs=3
  Mux2 : Mux  Inputs=2
  Mux3 : Mux  Inputs=2
  P0/ (Vo^np) : Gain  Gain=P0/(Mag_V0^np)  SaturateOnIntegerOverflow=on  OutDataTypeStr=Inherit: Same as input  ParamDataTypeStr=Inherit: Same as input
  PQ_ext : Constant  Value=PQext
  Product : Product  Inputs=/*  InputSameDT=on  SaturateOnIntegerOverflow=on  OutDataTypeStr=Inherit: Same as first input
  Q0/(Vo^nq) : Gain  Gain=Q0/(Mag_V0^nq)  SaturateOnIntegerOverflow=on  OutDataTypeStr=Inherit: Same as input  ParamDataTypeStr=Inherit: Same as input
  Real-Imag to Complex : RealImagToComplex
  Switch1 : Switch  Threshold=0.5  InputSameDT=on
  Switch3 : Switch  Threshold=Vmin  InputSameDT=on
  Switch4 : Switch  Threshold=Vmin  InputSameDT=on
  TF_P : Subsystem  mask(Transfer function){T1=Tp1, T2=Tp2, V_Init=P0}
      mask prompts: T1 "Time constant T1 (s):"; T2 "Time constant T2 (s):"; V_Init "Initial input and output :"
      mask help:
      | This block implements a continuous transfer function:
      |
      |          1+T1s
      | H(s)= ------
      |          1+T2s
      |
      | States are initialized according to  initial input and output value so that simulation starts in steady state.
      mask init:
      | numc=[T1 1];
      | denc=[T2 1];
      | [Ac,Bc,Cc,Dc]=tf2ss(numc,denc);
      | 
      | % Compute Initial states
      | I=eye(size(Ac));
      | x0c=inv(-Ac)*Bc*V_Init;
      mask Display: disp('1+T1s\n---\n1+T2s')
  TF_Q : Subsystem  mask(Transfer function){T1=Tq1, T2=Tq2, V_Init=Q0}
      mask prompts: T1 "Time constant T1 (s):"; T2 "Time constant T2 (s):"; V_Init "Initial input and output :"
      mask help:
      | This block implements a continuous transfer function:
      |
      |          1+T1s
      | H(s)= ------
      |          1+T2s
      |
      | States are initialized according to  initial input and output value so that simulation starts in steady state.
      mask init:
      | numc=[T1 1];
      | denc=[T2 1];
      | [Ac,Bc,Cc,Dc]=tf2ss(numc,denc);
      | 
      | % Compute Initial states
      | I=eye(size(Ac));
      | x0c=inv(-Ac)*Bc*V_Init;
      mask Display: disp('1+T1s\n---\n1+T2s')
  V^nq : Fcn  Expr=u[1]^u[2]
  V^nq , : Fcn  Expr=u[1]^u[2]
  Vmin^(np-2) : Gain  Gain=Vmin^(np-2)  SaturateOnIntegerOverflow=on  OutDataTypeStr=Inherit: Same as input  ParamDataTypeStr=Inherit: Same as input
  Vmin^(nq-2) : Gain  Gain=Vmin^(nq-2)  SaturateOnIntegerOverflow=on  OutDataTypeStr=Inherit: Same as input  ParamDataTypeStr=Inherit: Same as input
  np : Constant  Value=np
  nq : Constant  Value=nq
  pu>V : Gain  Gain=Vnom/sqrt(2)  SaturateOnIntegerOverflow=on  OutDataTypeStr=Inherit: Same as input  ParamDataTypeStr=Inherit: Same as input
  I1(A) : Outport  VectorParamsAs1DForOutWhenUnconnected=off
  VPQ : Outport  Port=2  VectorParamsAs1DForOutWhenUnconnected=off
  wires:
  TF_Q/1(Out1) -> Real-Imag to Complex/2
  TF_P/1(Out1) -> Real-Imag to Complex/1
  Complex to Real-Imag1/2 -> Mux1/3
  Complex to Real-Imag1/1 -> Mux1/2
  Mux1/1 -> VPQ/1
  Complex to Magnitude-Angle/1 -> Mux1/1, Switch4/2, Switch3/2, Mux2/1, Mux3/1, Math Function/1
  pu>V/1 -> Product/1
  PQ_ext/1 -> Switch1/2
  S_ext/1 -> Switch1/1
  Real-Imag to Complex/1 -> Switch1/3  "S_dyn"
  Switch1/1 -> Complex to Real-Imag1/1, Product/2  "S=P+jQ"
  Conj1/1 -> I1(A)/1
  Product/1 -> Conj1/1
  Switch4/1 -> Q0/(Vo^nq)/1
  P0/ (Vo^np)/1 -> TF_P/1(In1)
  Q0/(Vo^nq)/1 -> TF_Q/1(In1)
  Switch3/1 -> P0/ (Vo^np)/1
  np/1 -> Mux2/2
  Mux2/1 -> V^nq ,/1
  nq/1 -> Mux3/2
  Mux3/1 -> V^nq/1
  V1(pu)/1 -> pu>V/1, Complex to Magnitude-Angle/1
  V^nq/1 -> Switch4/1
  Math Function/1 -> Vmin^(np-2)/1, Vmin^(nq-2)/1
  Vmin^(np-2)/1 -> Switch3/3
  V^nq ,/1 -> Switch3/1
  Vmin^(nq-2)/1 -> Switch4/3

== system IEEE34_SPSload/SM_IEEE34/DL_808-810/Load B/model/Break Alg. Loop ==
  In : Inport
  Complex to Real-Imag : ComplexToRealImag
  Real-Imag to Complex : RealImagToComplex
  imag : simulink_extras/Additional Linear/Transfer Fcn (with initial outputs)  N=[1]  D="[100e-6  1]"  Y0=imag(I1_init*exp(-j*Pha_V0*pi/180))  U0=imag(I1_init*exp(-j*Pha_V0*pi/180))
  real : simulink_extras/Additional Linear/Transfer Fcn (with initial outputs)  N=[1]  D="[100e-6  1]"  Y0=real(I1_init*exp(-j*Pha_V0*pi/180))  U0=real(I1_init*exp(-j*Pha_V0*pi/180))
  Out : Outport  VectorParamsAs1DForOutWhenUnconnected=off
  wires:
  imag/1 -> Real-Imag to Complex/2
  Complex to Real-Imag/2 -> imag/1
  real/1 -> Real-Imag to Complex/1
  Complex to Real-Imag/1 -> real/1
  Real-Imag to Complex/1 -> Out/1
  In/1 -> Complex to Real-Imag/1

== system IEEE34_SPSload/SM_IEEE34/DL_808-810/Load B/model/PLL ==
  v (pu) : Inport
  freq (pu) : Inport  Port=2
  Gain : Gain  Gain=2*pi
  Gain1 : Gain  Gain=500
  Gain2 : Gain  Gain=freq
  IC : InitialCondition
  Integrator : Integrator
  Integrator1 : Integrator
  Product : Product  Inputs=**  RndMeth=Zero
  Sum1 : Sum  InputSameDT=on  SaturateOnIntegerOverflow=on  OutDataTypeStr=Inherit: Same as first input
  Trigonometric Function : Trigonometry  Operator=cos
  adaptive filter : Subsystem
  adaptive mean : Subsystem
  alpha (rad) : Outport  VectorParamsAs1DForOutWhenUnconnected=off
  wt : Outport  Port=2  VectorParamsAs1DForOutWhenUnconnected=off
  wires:
  freq (pu)/1 -> Gain2/1
  Gain2/1 -> adaptive filter/2(freq (Hz)), adaptive mean/2(freq (Hz)), Gain/1
  Trigonometric Function/1 -> Product/2
  adaptive mean/1(y) -> alpha (rad)/1
  Integrator1/1 -> Gain1/1
  Gain1/1 -> Sum1/1, adaptive mean/1(u)
  Sum1/1 -> Trigonometric Function/1
  Integrator/1 -> Sum1/2, wt/1
  Gain/1 -> Integrator/1
  adaptive filter/1(y) -> Integrator1/1
  Product/1 -> adaptive filter/1(u)
  v (pu)/1 -> IC/1
  IC/1 -> Product/1

== system IEEE34_SPSload/SM_IEEE34/DL_808-810/Load B/model/Positive Sequence current ==
  note: kp=Vmin^(np-2)/Vo^np
      | kq=Vmin^(nq-2)/Vo^nq
  note: V<Vmin
      | Constant impedance load :
      |
      |  P=Po*kp*V^2
      | Q=Qo*kq*V^2
  note: V>Vmin :
      |
      |    P=Po*(V/Vo)^np
      |    Q=Qo*(V/Vo)^np
  note: I1= (S/V1)'
  V1(pu) : Inport
  S_ext : Inport  Port=2
  Complex to Magnitude-Angle : ComplexToMagnitudeAngle  Output=Magnitude
  Complex to Real-Imag1 : ComplexToRealImag
  Conj1 : Math  Operator=conj  SignedPower=on  SaturateOnIntegerOverflow=on
  Math Function : Math  Operator=square  SignedPower=on  SaturateOnIntegerOverflow=on
  Mux1 : Mux  Inputs=3
  Mux2 : Mux  Inputs=2
  Mux3 : Mux  Inputs=2
  P0/ (Vo^np) : Gain  Gain=P0/(Mag_V0^np)  SaturateOnIntegerOverflow=on  OutDataTypeStr=Inherit: Same as input  ParamDataTypeStr=Inherit: Same as input
  PQ_ext : Constant  Value=PQext
  Product : Product  Inputs=/*  InputSameDT=on  SaturateOnIntegerOverflow=on  OutDataTypeStr=Inherit: Same as first input
  Q0/(Vo^nq) : Gain  Gain=Q0/(Mag_V0^nq)  SaturateOnIntegerOverflow=on  OutDataTypeStr=Inherit: Same as input  ParamDataTypeStr=Inherit: Same as input
  Real-Imag to Complex : RealImagToComplex
  Switch1 : Switch  Threshold=0.5  InputSameDT=on
  Switch3 : Switch  Threshold=Vmin  InputSameDT=on
  Switch4 : Switch  Threshold=Vmin  InputSameDT=on
  TF_P : Subsystem  mask(Transfer function){T1=Tp1, T2=Tp2, V_Init=P0}
      mask prompts: T1 "Time constant T1 (s):"; T2 "Time constant T2 (s):"; V_Init "Initial input and output :"
      mask help:
      | This block implements a continuous transfer function:
      |
      |          1+T1s
      | H(s)= ------
      |          1+T2s
      |
      | States are initialized according to  initial input and output value so that simulation starts in steady state.
      mask init:
      | numc=[T1 1];
      | denc=[T2 1];
      | [Ac,Bc,Cc,Dc]=tf2ss(numc,denc);
      | 
      | % Compute Initial states
      | I=eye(size(Ac));
      | x0c=inv(-Ac)*Bc*V_Init;
      mask Display: disp('1+T1s\n---\n1+T2s')
  TF_Q : Subsystem  mask(Transfer function){T1=Tq1, T2=Tq2, V_Init=Q0}
      mask prompts: T1 "Time constant T1 (s):"; T2 "Time constant T2 (s):"; V_Init "Initial input and output :"
      mask help:
      | This block implements a continuous transfer function:
      |
      |          1+T1s
      | H(s)= ------
      |          1+T2s
      |
      | States are initialized according to  initial input and output value so that simulation starts in steady state.
      mask init:
      | numc=[T1 1];
      | denc=[T2 1];
      | [Ac,Bc,Cc,Dc]=tf2ss(numc,denc);
      | 
      | % Compute Initial states
      | I=eye(size(Ac));
      | x0c=inv(-Ac)*Bc*V_Init;
      mask Display: disp('1+T1s\n---\n1+T2s')
  V^nq : Fcn  Expr=u[1]^u[2]
  V^nq , : Fcn  Expr=u[1]^u[2]
  Vmin^(np-2) : Gain  Gain=Vmin^(np-2)  SaturateOnIntegerOverflow=on  OutDataTypeStr=Inherit: Same as input  ParamDataTypeStr=Inherit: Same as input
  Vmin^(nq-2) : Gain  Gain=Vmin^(nq-2)  SaturateOnIntegerOverflow=on  OutDataTypeStr=Inherit: Same as input  ParamDataTypeStr=Inherit: Same as input
  np : Constant  Value=np
  nq : Constant  Value=nq
  pu>V : Gain  Gain=Vnom/sqrt(2)  SaturateOnIntegerOverflow=on  OutDataTypeStr=Inherit: Same as input  ParamDataTypeStr=Inherit: Same as input
  I1(A) : Outport  VectorParamsAs1DForOutWhenUnconnected=off
  VPQ : Outport  Port=2  VectorParamsAs1DForOutWhenUnconnected=off
  wires:
  Vmin^(nq-2)/1 -> Switch4/3
  V^nq ,/1 -> Switch3/1
  Vmin^(np-2)/1 -> Switch3/3
  Math Function/1 -> Vmin^(nq-2)/1, Vmin^(np-2)/1
  V^nq/1 -> Switch4/1
  V1(pu)/1 -> Complex to Magnitude-Angle/1, pu>V/1
  Mux3/1 -> V^nq/1
  nq/1 -> Mux3/2
  Mux2/1 -> V^nq ,/1
  np/1 -> Mux2/2
  Switch3/1 -> P0/ (Vo^np)/1
  Q0/(Vo^nq)/1 -> TF_Q/1(In1)
  P0/ (Vo^np)/1 -> TF_P/1(In1)
  Switch4/1 -> Q0/(Vo^nq)/1
  Product/1 -> Conj1/1
  Conj1/1 -> I1(A)/1
  Switch1/1 -> Product/2, Complex to Real-Imag1/1  "S=P+jQ"
  Real-Imag to Complex/1 -> Switch1/3  "S_dyn"
  S_ext/1 -> Switch1/1
  PQ_ext/1 -> Switch1/2
  pu>V/1 -> Product/1
  Complex to Magnitude-Angle/1 -> Math Function/1, Mux3/1, Mux2/1, Switch3/2, Switch4/2, Mux1/1
  Mux1/1 -> VPQ/1
  Complex to Real-Imag1/1 -> Mux1/2
  Complex to Real-Imag1/2 -> Mux1/3
  TF_P/1(Out1) -> Real-Imag to Complex/1
  TF_Q/1(Out1) -> Real-Imag to Complex/2

== system IEEE34_SPSload/SM_IEEE34/DL_816-1/Load B/model/Break Alg. Loop ==
  In : Inport
  Complex to Real-Imag : ComplexToRealImag
  Real-Imag to Complex : RealImagToComplex
  imag : simulink_extras/Additional Linear/Transfer Fcn (with initial outputs)  N=[1]  D="[100e-6  1]"  Y0=imag(I1_init*exp(-j*Pha_V0*pi/180))  U0=imag(I1_init*exp(-j*Pha_V0*pi/180))
  real : simulink_extras/Additional Linear/Transfer Fcn (with initial outputs)  N=[1]  D="[100e-6  1]"  Y0=real(I1_init*exp(-j*Pha_V0*pi/180))  U0=real(I1_init*exp(-j*Pha_V0*pi/180))
  Out : Outport  VectorParamsAs1DForOutWhenUnconnected=off
  wires:
  In/1 -> Complex to Real-Imag/1
  Real-Imag to Complex/1 -> Out/1
  Complex to Real-Imag/1 -> real/1
  real/1 -> Real-Imag to Complex/1
  Complex to Real-Imag/2 -> imag/1
  imag/1 -> Real-Imag to Complex/2

== system IEEE34_SPSload/SM_IEEE34/DL_816-1/Load B/model/PLL ==
  v (pu) : Inport
  freq (pu) : Inport  Port=2
  Gain : Gain  Gain=2*pi
  Gain1 : Gain  Gain=500
  Gain2 : Gain  Gain=freq
  IC : InitialCondition
  Integrator : Integrator
  Integrator1 : Integrator
  Product : Product  Inputs=**  RndMeth=Zero
  Sum1 : Sum  InputSameDT=on  SaturateOnIntegerOverflow=on  OutDataTypeStr=Inherit: Same as first input
  Trigonometric Function : Trigonometry  Operator=cos
  adaptive filter : Subsystem
  adaptive mean : Subsystem
  alpha (rad) : Outport  VectorParamsAs1DForOutWhenUnconnected=off
  wt : Outport  Port=2  VectorParamsAs1DForOutWhenUnconnected=off
  wires:
  IC/1 -> Product/1
  v (pu)/1 -> IC/1
  Product/1 -> adaptive filter/1(u)
  adaptive filter/1(y) -> Integrator1/1
  Gain/1 -> Integrator/1
  Integrator/1 -> wt/1, Sum1/2
  Sum1/1 -> Trigonometric Function/1
  Gain1/1 -> adaptive mean/1(u), Sum1/1
  Integrator1/1 -> Gain1/1
  adaptive mean/1(y) -> alpha (rad)/1
  Trigonometric Function/1 -> Product/2
  Gain2/1 -> Gain/1, adaptive mean/2(freq (Hz)), adaptive filter/2(freq (Hz))
  freq (pu)/1 -> Gain2/1

== system IEEE34_SPSload/SM_IEEE34/DL_816-1/Load B/model/Positive Sequence current ==
  note: I1= (S/V1)'
  note: V>Vmin :
      |
      |    P=Po*(V/Vo)^np
      |    Q=Qo*(V/Vo)^np
  note: V<Vmin
      | Constant impedance load :
      |
      |  P=Po*kp*V^2
      | Q=Qo*kq*V^2
  note: kp=Vmin^(np-2)/Vo^np
      | kq=Vmin^(nq-2)/Vo^nq
  V1(pu) : Inport
  S_ext : Inport  Port=2
  Complex to Magnitude-Angle : ComplexToMagnitudeAngle  Output=Magnitude
  Complex to Real-Imag1 : ComplexToRealImag
  Conj1 : Math  Operator=conj  SignedPower=on  SaturateOnIntegerOverflow=on
  Math Function : Math  Operator=square  SignedPower=on  SaturateOnIntegerOverflow=on
  Mux1 : Mux  Inputs=3
  Mux2 : Mux  Inputs=2
  Mux3 : Mux  Inputs=2
  P0/ (Vo^np) : Gain  Gain=P0/(Mag_V0^np)  SaturateOnIntegerOverflow=on  OutDataTypeStr=Inherit: Same as input  ParamDataTypeStr=Inherit: Same as input
  PQ_ext : Constant  Value=PQext
  Product : Product  Inputs=/*  InputSameDT=on  SaturateOnIntegerOverflow=on  OutDataTypeStr=Inherit: Same as first input
  Q0/(Vo^nq) : Gain  Gain=Q0/(Mag_V0^nq)  SaturateOnIntegerOverflow=on  OutDataTypeStr=Inherit: Same as input  ParamDataTypeStr=Inherit: Same as input
  Real-Imag to Complex : RealImagToComplex
  Switch1 : Switch  Threshold=0.5  InputSameDT=on
  Switch3 : Switch  Threshold=Vmin  InputSameDT=on
  Switch4 : Switch  Threshold=Vmin  InputSameDT=on
  TF_P : Subsystem  mask(Transfer function){T1=Tp1, T2=Tp2, V_Init=P0}
      mask prompts: T1 "Time constant T1 (s):"; T2 "Time constant T2 (s):"; V_Init "Initial input and output :"
      mask help:
      | This block implements a continuous transfer function:
      |
      |          1+T1s
      | H(s)= ------
      |          1+T2s
      |
      | States are initialized according to  initial input and output value so that simulation starts in steady state.
      mask init:
      | numc=[T1 1];
      | denc=[T2 1];
      | [Ac,Bc,Cc,Dc]=tf2ss(numc,denc);
      | 
      | % Compute Initial states
      | I=eye(size(Ac));
      | x0c=inv(-Ac)*Bc*V_Init;
      mask Display: disp('1+T1s\n---\n1+T2s')
  TF_Q : Subsystem  mask(Transfer function){T1=Tq1, T2=Tq2, V_Init=Q0}
      mask prompts: T1 "Time constant T1 (s):"; T2 "Time constant T2 (s):"; V_Init "Initial input and output :"
      mask help:
      | This block implements a continuous transfer function:
      |
      |          1+T1s
      | H(s)= ------
      |          1+T2s
      |
      | States are initialized according to  initial input and output value so that simulation starts in steady state.
      mask init:
      | numc=[T1 1];
      | denc=[T2 1];
      | [Ac,Bc,Cc,Dc]=tf2ss(numc,denc);
      | 
      | % Compute Initial states
      | I=eye(size(Ac));
      | x0c=inv(-Ac)*Bc*V_Init;
      mask Display: disp('1+T1s\n---\n1+T2s')
  V^nq : Fcn  Expr=u[1]^u[2]
  V^nq , : Fcn  Expr=u[1]^u[2]
  Vmin^(np-2) : Gain  Gain=Vmin^(np-2)  SaturateOnIntegerOverflow=on  OutDataTypeStr=Inherit: Same as input  ParamDataTypeStr=Inherit: Same as input
  Vmin^(nq-2) : Gain  Gain=Vmin^(nq-2)  SaturateOnIntegerOverflow=on  OutDataTypeStr=Inherit: Same as input  ParamDataTypeStr=Inherit: Same as input
  np : Constant  Value=np
  nq : Constant  Value=nq
  pu>V : Gain  Gain=Vnom/sqrt(2)  SaturateOnIntegerOverflow=on  OutDataTypeStr=Inherit: Same as input  ParamDataTypeStr=Inherit: Same as input
  I1(A) : Outport  VectorParamsAs1DForOutWhenUnconnected=off
  VPQ : Outport  Port=2  VectorParamsAs1DForOutWhenUnconnected=off
  wires:
  TF_Q/1(Out1) -> Real-Imag to Complex/2
  TF_P/1(Out1) -> Real-Imag to Complex/1
  Complex to Real-Imag1/2 -> Mux1/3
  Complex to Real-Imag1/1 -> Mux1/2
  Mux1/1 -> VPQ/1
  Complex to Magnitude-Angle/1 -> Mux1/1, Switch4/2, Switch3/2, Mux2/1, Mux3/1, Math Function/1
  pu>V/1 -> Product/1
  PQ_ext/1 -> Switch1/2
  S_ext/1 -> Switch1/1
  Real-Imag to Complex/1 -> Switch1/3  "S_dyn"
  Switch1/1 -> Complex to Real-Imag1/1, Product/2  "S=P+jQ"
  Conj1/1 -> I1(A)/1
  Product/1 -> Conj1/1
  Switch4/1 -> Q0/(Vo^nq)/1
  P0/ (Vo^np)/1 -> TF_P/1(In1)
  Q0/(Vo^nq)/1 -> TF_Q/1(In1)
  Switch3/1 -> P0/ (Vo^np)/1
  np/1 -> Mux2/2
  Mux2/1 -> V^nq ,/1
  nq/1 -> Mux3/2
  Mux3/1 -> V^nq/1
  V1(pu)/1 -> pu>V/1, Complex to Magnitude-Angle/1
  V^nq/1 -> Switch4/1
  Math Function/1 -> Vmin^(np-2)/1, Vmin^(nq-2)/1
  Vmin^(np-2)/1 -> Switch3/3
  V^nq ,/1 -> Switch3/1
  Vmin^(nq-2)/1 -> Switch4/3
